simulink model "Marine_LocoMotive_UAV_est_git"  (R2018a)
settings: Solver=ode4  StartTime=0.0  StopTime=40  FixedStep=T  MaxStep=2*T  MinStep=T  RelTol=1e-4
values from neighbouring files (symbols this model uses):
  a_11 = 0.05*m_b    (= 0.625)    [Marine_LocoMotive_UAV_est_git_parameters.m]    (also in Marine_LocoMotive_UAV_medium_est_git_parameters.m = 1.6875; heave_dynamics_chart.m)
  a_33 = m_b    (= 12.5)    [Marine_LocoMotive_UAV_est_git_parameters.m]    (also in Marine_LocoMotive_UAV_medium_est_git_parameters.m = 33.75; heave_dynamics_chart.m)
  A_w = 1*3.3/2    (= 1.65)    [Marine_LocoMotive_UAV_est_git_parameters.m]    (also in Marine_LocoMotive_UAV_medium_est_git_parameters.m = 0.6)
  A_w2 = 1*1.2/2    (= 0.6)    [Marine_LocoMotive_UAV_est_git_parameters.m]    (also in Marine_LocoMotive_UAV_medium_est_git_parameters.m = 0.305)
  Ac = 0.0331    [Marine_LocoMotive_UAV_est_git_parameters.m]    (also in Marine_LocoMotive_UAV_medium_est_git_parameters.m = 0.422)
  alpha_bar = pi/4    (= 0.785398163397)    [Marine_LocoMotive_UAV_est_git_parameters.m]    (also in Marine_LocoMotive_UAV_medium_est_git_parameters.m; heave_dynamics_chart.m = pi/4*sign(V_bar(j)))
  Am = sysd.denominator{1}    [Marine_LocoMotive_UAV_est_git_parameters.m]    (also in Marine_LocoMotive_UAV_medium_est_git_parameters.m)
  Am1_LPF = sysd.denominator{1}    [Marine_LocoMotive_UAV_est_git_parameters.m]    (also in Marine_LocoMotive_UAV_medium_est_git_parameters.m)
  Am2_LPF = sysd.denominator{1}    [Marine_LocoMotive_UAV_est_git_parameters.m]    (also in Marine_LocoMotive_UAV_medium_est_git_parameters.m)
  Am_asw_LPF = sysd.denominator{1}    [Marine_LocoMotive_UAV_est_git_parameters.m]    (also in Marine_LocoMotive_UAV_medium_est_git_parameters.m)
  Am_coup_LPF = sysd.denominator{1}    [Marine_LocoMotive_UAV_est_git_parameters.m]    (also in Marine_LocoMotive_UAV_medium_est_git_parameters.m)
  Am_fast_coup_LPF = sysd.denominator{1}    [Marine_LocoMotive_UAV_est_git_parameters.m]    (also in Marine_LocoMotive_UAV_medium_est_git_parameters.m)
  Am_rdeL_LPF = sysd.denominator{1}    [Marine_LocoMotive_UAV_est_git_parameters.m]    (also in Marine_LocoMotive_UAV_medium_est_git_parameters.m)
  Am_reL_LPF = sysd.denominator{1}    [Marine_LocoMotive_UAV_est_git_parameters.m]    (also in Marine_LocoMotive_UAV_medium_est_git_parameters.m)
  Am_rref20_LPF = sysd.denominator{1}    [Marine_LocoMotive_UAV_est_git_parameters.m]    (also in Marine_LocoMotive_UAV_medium_est_git_parameters.m)
  Am_rref_LPF = sysd.denominator{1}    [Marine_LocoMotive_UAV_est_git_parameters.m]    (also in Marine_LocoMotive_UAV_medium_est_git_parameters.m)
  AmAlpha_LPF = sysd.denominator{1}    [Marine_LocoMotive_UAV_est_git_parameters.m]    (also in Marine_LocoMotive_UAV_medium_est_git_parameters.m)
  Amp_sf = 3    [Marine_LocoMotive_UAV_est_git_parameters.m]    (also in Marine_LocoMotive_UAV_medium_est_git_parameters.m)
  Amp_sf_rp = 0.05*m_u*g    (= 0.8829)    [Marine_LocoMotive_UAV_est_git_parameters.m]    (also in Marine_LocoMotive_UAV_medium_est_git_parameters.m = 9.56475)
  AmV_LPF = sysd.denominator{1}    [Marine_LocoMotive_UAV_est_git_parameters.m]    (also in Marine_LocoMotive_UAV_medium_est_git_parameters.m)
  AmZ_LPF = sysd.denominator{1}    [Marine_LocoMotive_UAV_est_git_parameters.m]    (also in Marine_LocoMotive_UAV_medium_est_git_parameters.m)
  b_11 = 0    [Marine_LocoMotive_UAV_est_git_parameters.m]    (also in Marine_LocoMotive_UAV_medium_est_git_parameters.m; heave_dynamics_chart.m)
  b_33 = 2*m_b*omega_h    (= 19.6349540849)    [Marine_LocoMotive_UAV_est_git_parameters.m]    (also in Marine_LocoMotive_UAV_medium_est_git_parameters.m = 84.8230016469; buoyancy_calc.m = 4.18879020479; heave_dynamics_chart.m = 2*m_b*omega_h)
  Bm = sysd.numerator{1}    [Marine_LocoMotive_UAV_est_git_parameters.m]    (also in Marine_LocoMotive_UAV_medium_est_git_parameters.m)
  Bm1_LPF = sysd.numerator{1}    [Marine_LocoMotive_UAV_est_git_parameters.m]    (also in Marine_LocoMotive_UAV_medium_est_git_parameters.m)
  Bm2_LPF = sysd.numerator{1}    [Marine_LocoMotive_UAV_est_git_parameters.m]    (also in Marine_LocoMotive_UAV_medium_est_git_parameters.m)
  Bm_asw_LPF = sysd.numerator{1}    [Marine_LocoMotive_UAV_est_git_parameters.m]    (also in Marine_LocoMotive_UAV_medium_est_git_parameters.m)
  Bm_coup_LPF = sysd.numerator{1}    [Marine_LocoMotive_UAV_est_git_parameters.m]    (also in Marine_LocoMotive_UAV_medium_est_git_parameters.m)
  Bm_fast_coup_LPF = sysd.numerator{1}    [Marine_LocoMotive_UAV_est_git_parameters.m]    (also in Marine_LocoMotive_UAV_medium_est_git_parameters.m)
  Bm_rdeL_LPF = sysd.numerator{1}    [Marine_LocoMotive_UAV_est_git_parameters.m]    (also in Marine_LocoMotive_UAV_medium_est_git_parameters.m)
  Bm_reL_LPF = sysd.numerator{1}    [Marine_LocoMotive_UAV_est_git_parameters.m]    (also in Marine_LocoMotive_UAV_medium_est_git_parameters.m)
  Bm_rref20_LPF = sysd.numerator{1}    [Marine_LocoMotive_UAV_est_git_parameters.m]    (also in Marine_LocoMotive_UAV_medium_est_git_parameters.m)
  Bm_rref_LPF = sysd.numerator{1}    [Marine_LocoMotive_UAV_est_git_parameters.m]    (also in Marine_LocoMotive_UAV_medium_est_git_parameters.m)
  BmAlpha_LPF = sysd.numerator{1}    [Marine_LocoMotive_UAV_est_git_parameters.m]    (also in Marine_LocoMotive_UAV_medium_est_git_parameters.m)
  BmV_LPF = sysd.numerator{1}    [Marine_LocoMotive_UAV_est_git_parameters.m]    (also in Marine_LocoMotive_UAV_medium_est_git_parameters.m)
  BmZ_LPF = sysd.numerator{1}    [Marine_LocoMotive_UAV_est_git_parameters.m]    (also in Marine_LocoMotive_UAV_medium_est_git_parameters.m)
  C_S = [5;9]*10^-3    [Marine_LocoMotive_UAV_est_git_parameters.m]    (also in Marine_LocoMotive_UAV_medium_est_git_parameters.m; heave_dynamics_chart.m = 0.075/(log10(Re)-2)^2)
  Cd_u = 0.2    [Marine_LocoMotive_UAV_est_git_parameters.m]    (also in Marine_LocoMotive_UAV_medium_est_git_parameters.m)
  D_x = b_11 + D_s(1)    [Marine_LocoMotive_UAV_est_git_parameters.m]    (also in Marine_LocoMotive_UAV_medium_est_git_parameters.m; heave_dynamics_chart.m = b_11 + D_s(i,j))
  D_z = b_33 + D_s(2)    [Marine_LocoMotive_UAV_est_git_parameters.m]    (also in Marine_LocoMotive_UAV_medium_est_git_parameters.m; heave_dynamics_chart.m)
  dc_M_p = 6.7    [Marine_LocoMotive_UAV_est_git_parameters.m]    (also in Marine_LocoMotive_UAV_medium_est_git_parameters.m)
  Delta_h = (A_im/A_b-0.5)*h_b    (= -0.0625)    [Marine_LocoMotive_UAV_est_git_parameters.m]    (also in Marine_LocoMotive_UAV_medium_est_git_parameters.m = -0.075; heave_dynamics_chart.m)
  eps_V = 0.1    [Marine_LocoMotive_UAV_est_git_parameters.m]    (also in Marine_LocoMotive_UAV_medium_est_git_parameters.m)
  epsilon_1 = 5    [Marine_LocoMotive_UAV_est_git_parameters.m]    (also in Marine_LocoMotive_UAV_medium_est_git_parameters.m)
  epsilon_e_u1 = 0.05    [Marine_LocoMotive_UAV_est_git_parameters.m]    (also in Marine_LocoMotive_UAV_medium_est_git_parameters.m)
  epsilon_w = 0    [Marine_LocoMotive_UAV_est_git_parameters.m]    (also in Marine_LocoMotive_UAV_medium_est_git_parameters.m)
  epsilon_w2 = pi    (= 3.14159265359)    [Marine_LocoMotive_UAV_est_git_parameters.m]    (also in Marine_LocoMotive_UAV_medium_est_git_parameters.m)
  g = 9.81    [Marine_LocoMotive_UAV_est_git_parameters.m]    (also in Marine_LocoMotive_UAV_medium_est_git_parameters.m; heave_dynamics_chart.m)
  gamma_d_p = (2*0.3/0.03*2*0.2*12/4)/10    (= 2.4)    [Marine_LocoMotive_UAV_est_git_parameters.m]    (also in Marine_LocoMotive_UAV_medium_est_git_parameters.m)
  H = 10    [Marine_LocoMotive_UAV_est_git_parameters.m]    (also in Marine_LocoMotive_UAV_medium_est_git_parameters.m)
  h_b = 0.25    [Marine_LocoMotive_UAV_est_git_parameters.m]    (also in Marine_LocoMotive_UAV_medium_est_git_parameters.m = 0.3; buoyancy_calc.m = 0.15; heave_dynamics_chart.m)
  J_b = m_b*h_b*l_b/12    (= 0.208333333333)    [Marine_LocoMotive_UAV_est_git_parameters.m]    (also in Marine_LocoMotive_UAV_medium_est_git_parameters.m = 1.265625; heave_dynamics_chart.m)
  J_u = 0.03    [Marine_LocoMotive_UAV_est_git_parameters.m]    (also in Marine_LocoMotive_UAV_medium_est_git_parameters.m = 1.51708333333)
  K = 40    [Marine_LocoMotive_UAV_est_git_parameters.m]    (also in Marine_LocoMotive_UAV_medium_est_git_parameters.m = 83.3333333333)
  k3 = 24    [Marine_LocoMotive_UAV_est_git_parameters.m]    (also in Marine_LocoMotive_UAV_medium_est_git_parameters.m)
  k4 = 0.8    [Marine_LocoMotive_UAV_est_git_parameters.m]    (also in Marine_LocoMotive_UAV_medium_est_git_parameters.m)
  k_w = omega_w^2/g    (= 0.0628797426165)    [Marine_LocoMotive_UAV_est_git_parameters.m]    (also in Marine_LocoMotive_UAV_medium_est_git_parameters.m = 0.160972141098; heave_dynamics_chart.m = omega_w^2/g)
  k_w2 = omega_w2^2/g    (= 0.160972141098)    [Marine_LocoMotive_UAV_est_git_parameters.m]    (also in Marine_LocoMotive_UAV_medium_est_git_parameters.m = 0.251518970466)
  kd_a = 5.6    [Marine_LocoMotive_UAV_est_git_parameters.m]    (also in Marine_LocoMotive_UAV_medium_est_git_parameters.m)
  kd_r = 19.5    [Marine_LocoMotive_UAV_est_git_parameters.m]    (also in Marine_LocoMotive_UAV_medium_est_git_parameters.m)
  kd_t = 10    [Marine_LocoMotive_UAV_est_git_parameters.m]    (also in Marine_LocoMotive_UAV_medium_est_git_parameters.m = 25)
  kd_x = 5    [Marine_LocoMotive_UAV_est_git_parameters.m]    (also in Marine_LocoMotive_UAV_medium_est_git_parameters.m)
  kd_z = 2    [Marine_LocoMotive_UAV_est_git_parameters.m]    (also in Marine_LocoMotive_UAV_medium_est_git_parameters.m)
  ki_a = 1.6    [Marine_LocoMotive_UAV_est_git_parameters.m]    (also in Marine_LocoMotive_UAV_medium_est_git_parameters.m)
  ki_r = 9    [Marine_LocoMotive_UAV_est_git_parameters.m]    (also in Marine_LocoMotive_UAV_medium_est_git_parameters.m)
  ki_T = 12    [Marine_LocoMotive_UAV_est_git_parameters.m]    (also in Marine_LocoMotive_UAV_medium_est_git_parameters.m)
  ki_x = 1.2    [Marine_LocoMotive_UAV_est_git_parameters.m]    (also in Marine_LocoMotive_UAV_medium_est_git_parameters.m)
  ki_z = 1    [Marine_LocoMotive_UAV_est_git_parameters.m]    (also in Marine_LocoMotive_UAV_medium_est_git_parameters.m)
  kp_a = 9.6    [Marine_LocoMotive_UAV_est_git_parameters.m]    (also in Marine_LocoMotive_UAV_medium_est_git_parameters.m)
  kp_r = 45    [Marine_LocoMotive_UAV_est_git_parameters.m]    (also in Marine_LocoMotive_UAV_medium_est_git_parameters.m)
  kp_t = 20    [Marine_LocoMotive_UAV_est_git_parameters.m]    (also in Marine_LocoMotive_UAV_medium_est_git_parameters.m = 50)
  kp_T = 25    [Marine_LocoMotive_UAV_est_git_parameters.m]    (also in Marine_LocoMotive_UAV_medium_est_git_parameters.m)
  kp_x = 7    [Marine_LocoMotive_UAV_est_git_parameters.m]    (also in Marine_LocoMotive_UAV_medium_est_git_parameters.m)
  kp_z = 3    [Marine_LocoMotive_UAV_est_git_parameters.m]    (also in Marine_LocoMotive_UAV_medium_est_git_parameters.m)
  L = 0.2    [Marine_LocoMotive_UAV_est_git_parameters.m]    (also in Marine_LocoMotive_UAV_medium_est_git_parameters.m = 0.8)
  l_b = 0.8    [Marine_LocoMotive_UAV_est_git_parameters.m]    (also in Marine_LocoMotive_UAV_medium_est_git_parameters.m = 1.5; buoyancy_calc.m = 0.5; heave_dynamics_chart.m)
  Lc_0 = 7    [Marine_LocoMotive_UAV_est_git_parameters.m]    (also in Marine_LocoMotive_UAV_medium_est_git_parameters.m = 20)
  LIMIT_CMD_PITCH = 45*pi/180    (= 0.785398163397)    [Marine_LocoMotive_UAV_est_git_parameters.m]    (also in Marine_LocoMotive_UAV_medium_est_git_parameters.m)
  LIMIT_uCMD_HEIGHT = 0.9*n_motors*K    (= 144)    [Marine_LocoMotive_UAV_est_git_parameters.m]    (also in Marine_LocoMotive_UAV_medium_est_git_parameters.m = 450)
  m_b = rho_w*Vol_b/4    (= 12.5)    [Marine_LocoMotive_UAV_est_git_parameters.m]    (also in Marine_LocoMotive_UAV_medium_est_git_parameters.m = 33.75; buoyancy_calc.m = 5; heave_dynamics_chart.m)
  m_u = 1.8    [Marine_LocoMotive_UAV_est_git_parameters.m]    (also in Marine_LocoMotive_UAV_medium_est_git_parameters.m = 19.5)
  min_sf = 5    [Marine_LocoMotive_UAV_est_git_parameters.m]    (also in Marine_LocoMotive_UAV_medium_est_git_parameters.m)
  min_sf_rp = 0.35*m_u*g    (= 6.1803)    [Marine_LocoMotive_UAV_est_git_parameters.m]    (also in Marine_LocoMotive_UAV_medium_est_git_parameters.m = 66.95325)
  n_motors = 4    [Marine_LocoMotive_UAV_est_git_parameters.m]    (also in Marine_LocoMotive_UAV_medium_est_git_parameters.m = 6)
  nu_w = 1.787*10^-6    (= 1.787e-06)    [Marine_LocoMotive_UAV_est_git_parameters.m]    (also in Marine_LocoMotive_UAV_medium_est_git_parameters.m; buoyancy_calc.m; heave_dynamics_chart.m)
  omega_w = 2*pi/T_w    (= 0.785398163397)    [Marine_LocoMotive_UAV_est_git_parameters.m]    (also in Marine_LocoMotive_UAV_medium_est_git_parameters.m = 1.25663706144; heave_dynamics_chart.m = 2*pi/T_i)
  omega_w2 = 2*pi/T_w2    (= 1.25663706144)    [Marine_LocoMotive_UAV_est_git_parameters.m]    (also in Marine_LocoMotive_UAV_medium_est_git_parameters.m = 1.57079632679)
  r_0 = sqrt( (X0_b(1) - X0_u(1))^2 +(X0_b(2) - X0_u(2))^2 )    [Marine_LocoMotive_UAV_est_git_parameters.m]    (also in Marine_LocoMotive_UAV_medium_est_git_parameters.m)
  R_b = 0.1    [buoyancy_calc.m]
  r_bar = Lc_0-0.3    (= 6.7)    [Marine_LocoMotive_UAV_est_git_parameters.m]    (also in Marine_LocoMotive_UAV_medium_est_git_parameters.m = 19.7)
  r_min = (zu_bar-H)-0.2    [Marine_LocoMotive_UAV_est_git_parameters.m]    (also in Marine_LocoMotive_UAV_medium_est_git_parameters.m)
  rho_a = 1.225    [Marine_LocoMotive_UAV_est_git_parameters.m]    (also in Marine_LocoMotive_UAV_medium_est_git_parameters.m)
  rho_w = 1000    [Marine_LocoMotive_UAV_est_git_parameters.m]    (also in Marine_LocoMotive_UAV_medium_est_git_parameters.m; buoyancy_calc.m; heave_dynamics_chart.m)
  T = 1/500    (= 0.002)    [Marine_LocoMotive_UAV_est_git_parameters.m]    (also in Marine_LocoMotive_UAV_medium_est_git_parameters.m)
  T_init = 10    [Marine_LocoMotive_UAV_est_git_parameters.m]    (also in Marine_LocoMotive_UAV_medium_est_git_parameters.m)
  Theta0 = 0    [Marine_LocoMotive_UAV_est_git_parameters.m]    (also in Marine_LocoMotive_UAV_medium_est_git_parameters.m)
  torque_corr = 2*cosd(60)+1    [Marine_LocoMotive_UAV_est_git_parameters.m]    (also in Marine_LocoMotive_UAV_medium_est_git_parameters.m)
  u_s = w_dir*A_w^2*omega_w*k_w*exp(2*k_w*(-Delta_h/2))    [Marine_LocoMotive_UAV_est_git_parameters.m]    (also in Marine_LocoMotive_UAV_medium_est_git_parameters.m)
  u_s2 = w_dir2*A_w2^2*omega_w2*k_w2*exp(2*k_w2*(-Delta_h/2))    [Marine_LocoMotive_UAV_est_git_parameters.m]    (also in Marine_LocoMotive_UAV_medium_est_git_parameters.m)
  u_t = -1*0.5*1    (= -0.5)    [Marine_LocoMotive_UAV_est_git_parameters.m]    (also in Marine_LocoMotive_UAV_medium_est_git_parameters.m)
  u_w = 0*0.2    (= 0)    [Marine_LocoMotive_UAV_est_git_parameters.m]    (also in Marine_LocoMotive_UAV_medium_est_git_parameters.m)
  V0_b = [u_t+u_w+u_s+v_x_w, v_z_w].*[1 1]    [Marine_LocoMotive_UAV_est_git_parameters.m]    (also in Marine_LocoMotive_UAV_medium_est_git_parameters.m = [u_t+u_w+u_s+v_x_w, v_z_w])
  V0_u = V0_b    [Marine_LocoMotive_UAV_est_git_parameters.m]    (also in Marine_LocoMotive_UAV_medium_est_git_parameters.m = [0 0])
  V_bar = 4    [Marine_LocoMotive_UAV_est_git_parameters.m]    (also in Marine_LocoMotive_UAV_medium_est_git_parameters.m; heave_dynamics_chart.m = [-20:0.1:20]')
  Vol_b = A_b*l_b    (= 0.05)    [Marine_LocoMotive_UAV_est_git_parameters.m]    (also in Marine_LocoMotive_UAV_medium_est_git_parameters.m = 0.135; heave_dynamics_chart.m)
  w_dir = 1    [Marine_LocoMotive_UAV_est_git_parameters.m]    (also in Marine_LocoMotive_UAV_medium_est_git_parameters.m; heave_dynamics_chart.m)
  w_dir2 = 1    [Marine_LocoMotive_UAV_est_git_parameters.m]    (also in Marine_LocoMotive_UAV_medium_est_git_parameters.m)
  X0_b = [0,H-Delta_h]    [Marine_LocoMotive_UAV_est_git_parameters.m]    (also in Marine_LocoMotive_UAV_medium_est_git_parameters.m)
  X0_u = X0_b + [3/7 3/7]*Lc_0    [Marine_LocoMotive_UAV_est_git_parameters.m]    (also in Marine_LocoMotive_UAV_medium_est_git_parameters.m)
  zu_bar = X0_b(2) + Lc_0*sin(alpha_bar_0)    [Marine_LocoMotive_UAV_est_git_parameters.m]    (also in Marine_LocoMotive_UAV_medium_est_git_parameters.m)
undefined symbols (not defined in the file or in its folder): Am_HPF, Am_LPF, Am_LPF2, an1, an1_v, an2, an3, Bm_HPF, Bm_LPF, Bm_LPF2, bn1, bn1_v, bn2, bn3, DiscIntNeverNeededParam, F, Light, magnitude, MIL, OMEGA_FILTER_OUTER, Tc, Tg, Tn, Ts, Tsc, Tz, X_GPS_offset
libraries: simulink x55, simulink_extras x9, aerolibwind2 x2
(part 3 of 9)

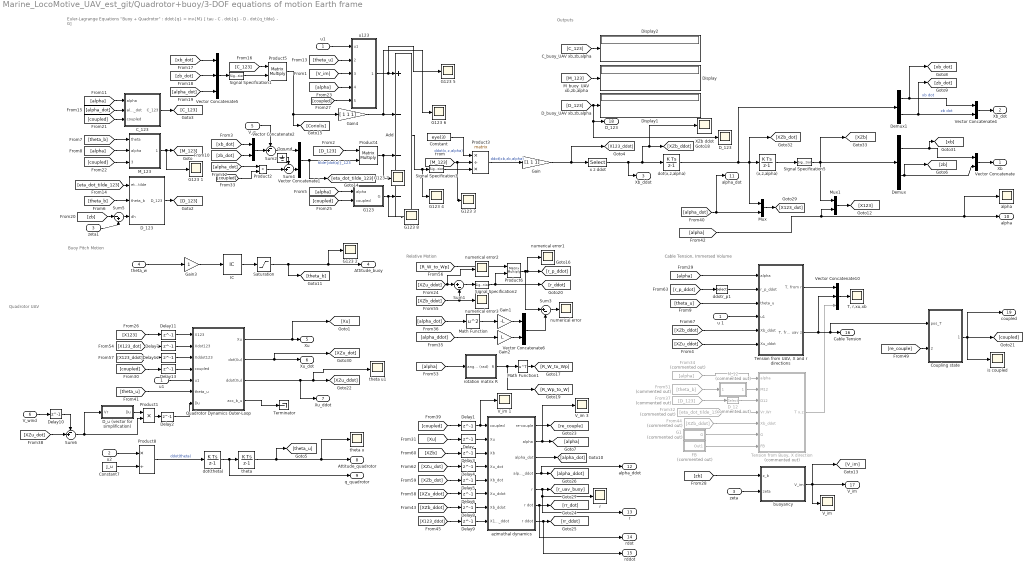
== system Marine_LocoMotive_UAV_est_git/Quadrotor+buoy/3-DOF equations of motion Earth frame ==
  note: Relative Motion
  note: Outputs
  note: Buoy Pitch Motion
  note: Cable Tension, Immersed Volume
  note: Quadrotor UAV
  note: Euler-Lagrange Equations "Buoy + Quadrotor" : ddot{q} = inv{M} [ tau - C . dot{q} - D . dot{q_tilde} - G]
  u1 : Inport
  u2 : Inport  Port=2
  zeta : Inport  Port=3
  theta_w : Inport  Port=4
  V_w : Inport  Port=5
  V_wind : Inport  Port=6
  "  r   " : Scope
  (x,z,alpha) : DiscreteIntegrator  InitialCondition=[pos_b_ini]  SampleTime=-1  ICPrevOutput=DiscIntNeverNeededParam  ICPrevScaledInput=DiscIntNeverNeededParam
  Add : Sum  Inputs=+---
  C_123 : Subsystem
  Constant : Constant  Value=eye(3)
  Constant7 : Constant  Value=J_u
  Coupling state : Subsystem
  D_12 : Selector  Commented=on  NumberOfDimensions=2  InputPortWidth=3  IndexOptions=Starting index (dialog),Starting index (dialog)  Indices=1,1  OutputSizes=2,2
  D_123 : Subsystem
  "D_123   " : Scope
  D_u (vector for simplification) : Subsystem
  Delay{,1,3..9,11..13} (12 alike) : Delay  DelayLength=1
  Delay10 : Delay  DelayLength=1  InitialCondition=[0 0]
  Delay2 : Delay  DelayLength=1  InitialCondition=[0 0]
  Demux : Demux  Outputs=2
  Demux1 : Demux  Outputs=2
  Display : Display
  Display1 : Display
  Display2 : Display
  FB : Subsystem  Commented=on
  From32 : From  Commented=on  GotoTag=eta_dot_tilde_12
  From34 : From  Commented=on  GotoTag=alpha
  From37 : From  Commented=on  GotoTag=D_123
  From44 : From  Commented=on  GotoTag=XZb_ddot
  From51 : From  Commented=on  GotoTag=theta_b
  G1 : Subsystem  Commented=on
  G123 : Subsystem
  G123 {1..8} (8 alike) : Scope
  Gain : Gain  Gain=[1 1 1]
  Gain1 : Gain  Gain=-L
  Gain2 : Gain  Gain=L
  Gain3 : Gain
  Gain4 : Gain  Gain=[ 1 1 1]
  Ground : Ground
  IC : InitialCondition  Value=0
  M_12 : Subsystem  Commented=on
  M_123 : Subsystem
  Math Function : Math  Operator=square  SaturateOnIntegerOverflow=on
  Math Function1 : Math  Operator=transpose  SaturateOnIntegerOverflow=on
  Mux : Mux  Inputs=2
  Mux1 : Mux  Inputs=2
  Product1 : Product  Inputs=**  SaturateOnIntegerOverflow=on  InputSameDT=on  OutDataTypeStr=Inherit: Same as first input
  Product2 : Product  Inputs=**  SaturateOnIntegerOverflow=on  InputSameDT=on  OutDataTypeStr=Inherit: Same as first input
  Product3 : Product  Inputs=*/*  Multiplication=Matrix(*)  SaturateOnIntegerOverflow=on  InputSameDT=on  OutDataTypeStr=Inherit: Same as first input
  Product4 : Product  Inputs=**  Multiplication=Matrix(*)  SaturateOnIntegerOverflow=on  InputSameDT=on  OutDataTypeStr=Inherit: Same as first input
  Product5 : Product  Inputs=**  Multiplication=Matrix(*)  SaturateOnIntegerOverflow=on  InputSameDT=on  OutDataTypeStr=Inherit: Same as first input
  Product6 : Product  Multiplication=Matrix(*)
  Product8 : Product  Inputs=*/  SaturateOnIntegerOverflow=on  InputSameDT=on  OutDataTypeStr=Inherit: Same as first input
  Quadrotor Dynamics Outer-Loop : Subsystem
  Saturation : Saturate  UpperLimit=0.15  LowerLimit=-0.15
  Signal Specification1 : SignalSpecification  Dimensions=3
  Signal Specification2 : SignalSpecification  Dimensions=2
  Signal Specification3 : SignalSpecification  Dimensions=3
  Signal Specification5 : SignalSpecification  Dimensions=2
  Sum1 : Sum  Inputs=|+-
  Sum2 : Sum  Inputs=-+|  SaturateOnIntegerOverflow=on
  Sum3 : Sum  Inputs=|+-
  Sum4 : Sum  Inputs=-+|  SaturateOnIntegerOverflow=on
  Sum5 : Sum  Inputs=|-+  SaturateOnIntegerOverflow=on
  Sum6 : Sum  Inputs=-+|  SaturateOnIntegerOverflow=on
  "T, r,xu,xb" : Scope
  "Tension from Buoy, X direction" : Subsystem  Commented=on
  "Tension from UAV, X and r directions" : Subsystem
  Terminator : Terminator
  "V_im " : Scope
  V_im 1 : Scope
  V_im 3 : Scope
  Vector Concatenate{,1..2,4,6} (5 alike) : Concatenate
  Vector Concatenate10 : Concatenate  NumInputs=3
  Vector Concatenate5 : Concatenate  NumInputs=3
  "XZb ddot " : Scope
  "alpha  " : Scope
  azimuthal dynamics : Subsystem
  buoyancy : Subsystem
  ddotr_p1 : Selector  InputPortWidth=2  IndexOptions=Index vector (dialog)  Indices=1  OutputSizes=2
  dot(theta) : DiscreteIntegrator  gainval=1  InitialCondition=q_b_ini  SampleTime=-1  ICPrevOutput=DiscIntNeverNeededParam  ICPrevScaledInput=DiscIntNeverNeededParam
  dot(x,z,alpha) : DiscreteIntegrator  InitialCondition=[v_b_ini]  SampleTime=-1  ICPrevOutput=DiscIntNeverNeededParam  ICPrevScaledInput=DiscIntNeverNeededParam
  "is coupled " : Scope
  numerical error{,1..3} (4 alike) : Scope
  "rotation matrix R " : Subsystem
  theta : DiscreteIntegrator  InitialCondition=theta_q_ini  SampleTime=-1  StateName=theta  ICPrevOutput=DiscIntNeverNeededParam  ICPrevScaledInput=DiscIntNeverNeededParam
  theta u : Scope
  theta u1 : Scope
  u 1 : InportShadow
  "u1  " : InportShadow
  u123 : Subsystem
  x z ddot : Selector  InputPortWidth=3  IndexOptions=Index vector (dialog)  Indices=[1 2]  OutputSizes=1
  zeta1 : InportShadow  Port=3
  Xb : Outport  Unit=m  InitialOutput=0
  Xb_dot : Outport  Port=2  Unit=m  InitialOutput=0
  Xb_ddot : Outport  Port=3  Unit=m  InitialOutput=0
  Attitude_buoy : Outport  Port=4  Unit=rad/s^2  InitialOutput=0
  Xu : Outport  Port=5  Unit=m  InitialOutput=0
  Xu_dot : Outport  Port=6  Unit=m/s  InitialOutput=0
  Xu_ddot : Outport  Port=7  Unit=m/s  InitialOutput=0
  Attitude_quadrotor : Outport  Port=8  Unit=rad  InitialOutput=0
  q_quadrotor : Outport  Port=9  Unit=rad/s  InitialOutput=0
  alpha : Outport  Port=10  Unit=m  InitialOutput=0
  alpha_dot : Outport  Port=11  Unit=m  InitialOutput=0
  alpha_ddot : Outport  Port=12  Unit=m  InitialOutput=0
  "  r" : Outport  Port=13  Unit=m  InitialOutput=0
  "  rdot" : Outport  Port=14  Unit=m  InitialOutput=0
  "  rddot" : Outport  Port=15  Unit=m  InitialOutput=0
  Cable Tension : Outport  Port=16  Unit=rad/s^2  InitialOutput=0
  V_im : Outport  Port=17  Unit=m  InitialOutput=0
  "D_123 " : Outport  Port=18  Unit=m  InitialOutput=0
  coupled : Outport  Port=19  Unit=m  InitialOutput=0
  wires:
  u123/1(u123) -> G123 5/1, Add/1
  Product4/1 -> G123 7/1, Add/3
  [D_123] -> Product4/1
  Vector Concatenate1/1 -> [eta_dot_tilde_123], Product4/2  "tilde{dot(q)}_123"
  G123/1(G) -> G123 8/1, Add/4
  [alpha] -> Mux1/2, "alpha  "/1, alpha/1
  [theta_b] -> D_123/2(theta_b)
  D_123/1(D_123) -> [D_123]
  [theta_b] -> M_123/1(theta)
  [alpha] -> M_123/2(alpha)
  Demux1/2 -> [zb_dot], Vector Concatenate4/2  "zb dot"
  Demux1/1 -> [xb_dot], Vector Concatenate4/1  "xb dot"
  [xb_dot] -> Vector Concatenate2/1
  [zb_dot] -> Vector Concatenate2/2
  Vector Concatenate2/1 -> Sum2/2
  V_w/1 -> Sum2/1
  Sum2/1 -> Vector Concatenate1/1
  Sum4/1 -> Vector Concatenate1/2
  theta_w/1 -> Gain3/1
  dot(theta)/1 -> q_quadrotor/1, theta/1
  theta/1 -> [theta_u], theta u/1, Attitude_quadrotor/1
  Constant7/1 -> Product8/2
  u2/1 -> Product8/1
  [theta_u] -> u123/2(theta)
  [V_im] -> u123/3(V_im)
  [alpha] -> G123/1(alpha)
  Demux/1 -> [xb], Vector Concatenate/1
  Demux/2 -> [zb], Vector Concatenate/2
  M_123/1(M_123) -> G123 1/1, [M_123]
  Product8/1 -> dot(theta)/1  "ddot(theta)"
  [M_123] -> G123 3/1, Product3/2
  Constant/1 -> Product3/1  "ddot(x,z,alpha)"
  Product3/1 -> Gain/1  "ddot(xb,zb,alpha)"
  IC/1 -> Saturation/1
  [alpha] -> C_123/1("alpha ")
  [alpha_dot] -> C_123/2(alpha_dot)
  C_123/1(C_123) -> [C_123]
  Vector Concatenate5/1 -> Signal Specification1/1
  [xb_dot] -> Vector Concatenate5/1
  [zb_dot] -> Vector Concatenate5/2
  [alpha_dot] -> Vector Concatenate5/3
  [C_123] -> Product5/1
  Product5/1 -> [Coriolis], Gain4/1
  Gain/1 -> [X123_ddot], x z ddot/1
  [alpha] -> u123/4(alpha)
  [r_p_ddot] -> ddotr_p1/1
  [theta_u] -> "Tension from UAV, X and r directions"/3(theta_u)
  u 1/1 -> "Tension from UAV, X and r directions"/4(u1)
  [D_123] -> "D_123 "/1, "D_123   "/1, Display1/1
  [M_123] -> Display/1
  [C_123] -> Display2/1
  (x,z,alpha)/1 -> Signal Specification5/1
  [zb] -> buoyancy/1(z_b)
  zeta/1 -> buoyancy/2(zeta)
  From34/1 -> "Tension from Buoy, X direction"/1(alpha)
  D_12/1 -> "Tension from Buoy, X direction"/3(D12)
  buoyancy/1(V_im) -> "V_im "/1, V_im/1, [V_im]
  M_12/1(M_12) -> "Tension from Buoy, X direction"/2(M12)
  From37/1 -> D_12/1
  From44/1 -> "Tension from Buoy, X direction"/5(Xb_ddot)
  From32/1 -> "Tension from Buoy, X direction"/4(Vr,Wr)
  [XZb_ddot] -> "Tension from UAV, X and r directions"/5(Xb_ddot)
  G1/1(G) -> "Tension from Buoy, X direction"/6(G)
  From51/1 -> M_12/1(theta)
  x z ddot/1 -> Xb_ddot/1, "XZb ddot "/1, [XZb_ddot], dot(x,z,alpha)/1
  ddotr_p1/1 -> "Tension from UAV, X and r directions"/2(r_p_ddot)
  [XZu_ddot] -> "Tension from UAV, X and r directions"/6(Xu_ddot)
  FB/1(Out1) -> "Tension from Buoy, X direction"/7(FB)
  Vector Concatenate10/1 -> "T, r,xu,xb"/1
  "Tension from Buoy, X direction"/1(T x,z) -> Vector Concatenate10/3
  Gain2/1 -> Vector Concatenate6/2
  [R_W_to_Wp] -> Product6/1
  Vector Concatenate6/1 -> Sum3/2
  "rotation matrix R "/1(R) -> [R_Wp_to_W], Math Function1/1
  Product6/1 -> Sum3/1, numerical error1/1, [r_p_ddot]
  Gain1/1 -> Vector Concatenate6/1
  Math Function/1 -> Gain1/1
  Sum1/1 -> Signal Specification2/1
  [XZu_ddot] -> numerical error2/1, Sum1/1
  Math Function1/1 -> [R_W_to_Wp]
  Sum3/1 -> numerical error/1
  [XZb_ddot] -> numerical error3/1, Sum1/2
  [alpha] -> "rotation matrix R "/1(angle (rad))
  [alpha_dot] -> Math Function/1
  Saturation/1 -> G123 2/1, Attitude_buoy/1, [theta_b]
  Add/1 -> G123 4/1, Signal Specification3/1
  Gain3/1 -> IC/1
  Gain4/1 -> G123 6/1, Add/2
  Product2/1 -> Sum4/2
  Ground/1 -> Sum4/1
  [eta_dot_tilde_123] -> D_123/1(eta_dot_tilde)
  Sum5/1 -> D_123/3(dh)
  [zb] -> Sum5/1
  zeta1/1 -> Sum5/2
  [coupled] -> C_123/3(coupled)
  [coupled] -> M_123/3(coupled)
  [coupled] -> G123/2(coupled)
  u1/1 -> u123/1(u1)
  Signal Specification1/1 -> Product5/2
  Signal Specification2/1 -> Product6/2, [r_ddot]
  Signal Specification3/1 -> Product3/3
  Signal Specification5/1 -> [XZb], Mux1/1, Demux/1
  Quadrotor Dynamics Outer-Loop/1(Xu) -> Xu/1, [Xu]
  [coupled] -> Delay13/1
  "u1  "/1 -> Quadrotor Dynamics Outer-Loop/5(u1)
  [theta_u] -> Quadrotor Dynamics Outer-Loop/6(theta_u)
  Quadrotor Dynamics Outer-Loop/2(dot(Xu)) -> [XZu_dot], Xu_dot/1
  Product1/1 -> Delay2/1
  [coupled] -> u123/5(coupled)
  [alpha_dot] -> Product2/1
  [coupled] -> Product2/2
  [Xu] -> Delay/1
  azimuthal dynamics/1(re-couple) -> [re_couple]
  azimuthal dynamics/2(alpha) -> V_im 3/1, [alpha]
  azimuthal dynamics/3("alpha_dot ") -> [alpha_dot]
  azimuthal dynamics/4(alpha_ddot) -> alpha_ddot/1, [alpha_ddot]
  Delay/1 -> azimuthal dynamics/2(Xu)
  azimuthal dynamics/5("r ") -> "  r"/1, "  r   "/1, [r_uav_buoy]
  [X123] -> Delay11/1
  Delay3/1 -> azimuthal dynamics/3(Xb)
  [X123_ddot] -> Delay12/1
  [X123_dot] -> Delay7/1
  dot(x,z,alpha)/1 -> Mux/1, (x,z,alpha)/1, [XZb_dot], Demux1/1
  [alpha_dot] -> alpha_dot/1, Mux/2
  Mux/1 -> [X123_dot]
  Mux1/1 -> [X123]
  Vector Concatenate4/1 -> Xb_dot/1
  Vector Concatenate/1 -> Xb/1
  [alpha] -> "Tension from UAV, X and r directions"/1(alpha)
  [XZb] -> Delay3/1
  [XZu_dot] -> Delay4/1
  [XZb_dot] -> Delay5/1
  [XZu_ddot] -> Delay6/1
  [XZb_ddot] -> Delay8/1
  [alpha_ddot] -> Gain2/1
  Delay4/1 -> azimuthal dynamics/4("Xu_dot ")
  [X123_ddot] -> Delay9/1
  Delay5/1 -> azimuthal dynamics/5(Xb_dot)
  Delay6/1 -> azimuthal dynamics/6(Xu_ddot)
  Delay8/1 -> azimuthal dynamics/7("Xb_ddot   ")
  Delay9/1 -> azimuthal dynamics/8("X123_ddot  ")
  [coupled] -> Delay1/1
  Delay1/1 -> V_im 1/1, azimuthal dynamics/1(coupled)
  Delay11/1 -> Quadrotor Dynamics Outer-Loop/1(X123)
  Delay12/1 -> Quadrotor Dynamics Outer-Loop/3(Xddot123)
  Delay7/1 -> Quadrotor Dynamics Outer-Loop/2(Xdot123)
  Delay13/1 -> Quadrotor Dynamics Outer-Loop/4(coupled)
  azimuthal dynamics/6(r dot) -> "  rdot"/1, [rr_dot]
  azimuthal dynamics/7(r ddot) -> "  rddot"/1, [rr_ddot]
  "Tension from UAV, X and r directions"/2("T, from uav z") -> Coupling state/1(pos_T), Cable Tension/1, Vector Concatenate10/2
  [re_couple] -> Coupling state/2(re_couple)
  Coupling state/1(is coupled) -> "is coupled "/1, coupled/1, [coupled]
  Quadrotor Dynamics Outer-Loop/3(ddot(Xu)) -> Xu_ddot/1, theta u1/1, [XZu_ddot]
  Quadrotor Dynamics Outer-Loop/4(acc_b_u) -> Terminator/1
  "Tension from UAV, X and r directions"/1("T, from r") -> Vector Concatenate10/1
  D_u (vector for simplification)/1(Du) -> Product1/1
  [XZu_dot] -> Sum6/2
  Sum6/1 -> D_u (vector for simplification)/1(Vr), Product1/2
  Delay2/1 -> Quadrotor Dynamics Outer-Loop/7(Du)
  V_wind/1 -> Delay10/1
  Delay10/1 -> Sum6/1

== system Marine_LocoMotive_UAV_est_git/Save to file/mean absolute error ==
  In1 : Inport
  Abs : Abs
  Add : Sum
  Constant : Constant  Value=T
  Delay : Delay  DelayLength=1
  IC : InitialCondition
  Product1 : Product  Inputs=*/
  Product2 : Product  Inputs=*/
  Out1 : Outport
  wires:
  Product2/1 -> IC/1
  Add/1 -> Product1/1, Delay/1
  Delay/1 -> Add/1
  [time] -> Product2/1
  In1/1 -> Abs/1
  Product1/1 -> Out1/1
  Constant/1 -> Product2/2
  IC/1 -> Product1/2
  Abs/1 -> Add/2

== system Marine_LocoMotive_UAV_est_git/Scope/Subsystem ==
  In1 : Inport
  In2 : Inport  Port=2
  Product : Product
  Sqrt : Sqrt  SaturateOnIntegerOverflow=on
  Subtract : Sum  Inputs=+-
  Sum of Elements : Sum  Inputs=+
  Out1 : Outport
  wires:
  In1/1 -> Subtract/2
  Product/1 -> Sum of Elements/1
  Subtract/1 -> Product/2, Product/1
  In2/1 -> Subtract/1
  Sqrt/1 -> Out1/1, [r]
  Sum of Elements/1 -> Sqrt/1

== system Marine_LocoMotive_UAV_est_git/Scope/absolute mean ==
  u : Inport
  Abs : Abs
  Bias : Bias  Bias=1/1000
  Clock : Clock
  Current velocity : Scope
  Current velocity1 : Scope
  Current velocity2 : Scope
  Discrete-Time Integrator : DiscreteIntegrator  gainval=1  SampleTime=T  ICPrevOutput=DiscIntNeverNeededParam  ICPrevScaledInput=DiscIntNeverNeededParam
  Divide1 : Product  Inputs=*/
  mean : Outport
  wires:
  Discrete-Time Integrator/1 -> Current velocity1/1, Divide1/1
  Abs/1 -> Discrete-Time Integrator/1
  u/1 -> Current velocity/1, Abs/1
  Divide1/1 -> mean/1
  Clock/1 -> Bias/1
  Bias/1 -> Current velocity2/1, Divide1/2

== system Marine_LocoMotive_UAV_est_git/Scope/absolute mean1 ==
  u : Inport
  Abs : Abs
  Bias : Bias  Bias=1/1000
  Clock : Clock
  Current velocity : Scope
  Current velocity1 : Scope
  Current velocity2 : Scope
  Discrete-Time Integrator : DiscreteIntegrator  gainval=1  SampleTime=T  ICPrevOutput=DiscIntNeverNeededParam  ICPrevScaledInput=DiscIntNeverNeededParam
  Divide1 : Product  Inputs=*/
  mean : Outport
  wires:
  Clock/1 -> Bias/1
  Divide1/1 -> mean/1
  u/1 -> Abs/1, Current velocity/1
  Abs/1 -> Discrete-Time Integrator/1
  Discrete-Time Integrator/1 -> Divide1/1, Current velocity1/1
  Bias/1 -> Divide1/2, Current velocity2/1

== system Marine_LocoMotive_UAV_est_git/Sea2/Single Wave ==
  note: Aw.Sin
  time : Inport
  x(t) : Inport  Port=2
  Constant : Constant  Value=epsilon
  Gain : Gain  Gain=omega
  Gain1 : Gain  Gain=k
  Gain2 : Gain  Gain=A
  Gain3 : Gain  Gain=omega*A
  Gain4 : Gain  Gain=omega*A
  Gain5 : Gain  Gain=A*k
  Sum : Sum  Inputs=++-
  Trigonometric Function : Trigonometry  Operator=sincos
  Trigonometric Function1 : Trigonometry  Operator=atan
  direction : Gain  Gain=w_dir
  direction1 : Gain  Gain=w_dir
  direction2 : Gain  Gain=w_dir
  zeta(x,t) : Outport
  theta_w(x,t) : Outport  Port=2
  u(z0,x,t) : Outport  Port=3
  w(z0,x,t) : Outport  Port=4
  wires:
  Gain/1 -> Sum/2
  Gain1/1 -> Sum/3
  x(t)/1 -> Gain1/1
  Trigonometric Function/1 -> Gain3/1, Gain2/1
  Constant/1 -> Sum/1
  time/1 -> direction/1
  direction/1 -> Gain/1
  Gain2/1 -> zeta(x,t)/1  "zeta(x,t)"
  Trigonometric Function/2 -> Gain5/1, Gain4/1
  Sum/1 -> Trigonometric Function/1
  Trigonometric Function1/1 -> theta_w(x,t)/1
  Gain5/1 -> Trigonometric Function1/1
  Gain3/1 -> direction1/1
  Gain4/1 -> direction2/1
  direction1/1 -> u(z0,x,t)/1
  direction2/1 -> w(z0,x,t)/1

== system Marine_LocoMotive_UAV_est_git/Sea2/Single Wave1 ==
  note: Aw.Sin
  time : Inport
  x(t) : Inport  Port=2
  Constant : Constant  Value=epsilon
  Gain : Gain  Gain=omega
  Gain1 : Gain  Gain=k
  Gain2 : Gain  Gain=A
  Gain3 : Gain  Gain=omega*A
  Gain4 : Gain  Gain=omega*A
  Gain5 : Gain  Gain=A*k
  Sum : Sum  Inputs=++-
  Trigonometric Function : Trigonometry  Operator=sincos
  Trigonometric Function1 : Trigonometry  Operator=atan
  direction : Gain  Gain=w_dir
  direction1 : Gain  Gain=w_dir
  direction2 : Gain  Gain=w_dir
  zeta(x,t) : Outport
  theta_w(x,t) : Outport  Port=2
  u(z0,x,t) : Outport  Port=3
  w(z0,x,t) : Outport  Port=4
  wires:
  direction2/1 -> w(z0,x,t)/1
  direction1/1 -> u(z0,x,t)/1
  Gain4/1 -> direction2/1
  Gain3/1 -> direction1/1
  Gain5/1 -> Trigonometric Function1/1
  Trigonometric Function1/1 -> theta_w(x,t)/1
  Sum/1 -> Trigonometric Function/1
  Trigonometric Function/2 -> Gain4/1, Gain5/1
  Gain2/1 -> zeta(x,t)/1  "zeta(x,t)"
  direction/1 -> Gain/1
  time/1 -> direction/1
  Constant/1 -> Sum/1
  Trigonometric Function/1 -> Gain2/1, Gain3/1
  x(t)/1 -> Gain1/1
  Gain1/1 -> Sum/3
  Gain/1 -> Sum/2

== system Marine_LocoMotive_UAV_est_git/Sea2/Theta_water surface (two waves) ==
  w1 : Inport
  w2 : Inport  Port=2
  Gain2 : Gain  Gain=1/(omega_w)
  Gain3 : Gain  Gain=k_w
  Gain4 : Gain  Gain=1/(omega_w2)
  Gain5 : Gain  Gain=k_w2
  Sum2 : Sum  Inputs=++|
  direction1 : Gain  Gain=1/w_dir
  direction2 : Gain  Gain=1/w_dir2
  Out1 : Outport
  wires:
  Gain4/1 -> direction2/1
  direction2/1 -> Gain5/1
  Sum2/1 -> Out1/1
  w1/1 -> Gain2/1
  Gain3/1 -> Sum2/1
  Gain5/1 -> Sum2/2
  w2/1 -> Gain4/1
  direction1/1 -> Gain3/1
  Gain2/1 -> direction1/1

== system Marine_LocoMotive_UAV_est_git/Sensors and Filters/Coupling detection by r ==
  In1 : Inport
  In2 : Inport  Port=2
  Constant1 : Constant  Value=0
  Coupling state : Subsystem
  Data Type Conversion : DataTypeConversion  OutDataTypeStr=double
  IC2 : InitialCondition  Value=0
  Switch14 : Switch  Criteria=u2 > Threshold  Threshold=0.5
  cable length with safety margine : simulink/Logic and Bit Operations/Compare To Constant  relop=>=  const=Lc_0+0.005  OutDataTypeStr=boolean
  is coupled {,2..4} (4 alike) : Scope
  is coupled : Outport
  wires:
  IC2/1 -> Switch14/3
  In1/1 -> is coupled 3/1, Coupling state/1(r_est), is coupled 2/1, cable length with safety margine/1
  Switch14/1 -> [re_couple]
  cable length with safety margine/1 -> is coupled 4/1, Data Type Conversion/1
  [re_couple] -> Coupling state/2(re_couple)
  Data Type Conversion/1 -> IC2/1
  Coupling state/1(is coupled) -> is coupled/1, "is coupled "/1
  Constant1/1 -> Switch14/1
  In2/1 -> Switch14/2

== system Marine_LocoMotive_UAV_est_git/Sensors and Filters/Data processing ==
  Acc : Inport
  "GPS " : Inport  Port=2
  p,q,r : Inport  Port=3
  Sonar : Inport  Port=4
  Estimate Attitude : Subsystem  TreatAsAtomicUnit=on  SystemSampleTime=Tc
  Estimate Position : Subsystem  TreatAsAtomicUnit=on  SystemSampleTime=Tc
  "Euler " : Selector  InputPortWidth=5  IndexOptions=Index vector (dialog)  Indices=[3]  OutputSizes=1
  GPS : InportShadow  Port=2
  Xe_est : Outport
  Ve_est : Outport  Port=2
  q_gyro : Outport  Port=3
  "q_est " : Outport  Port=4
  pitch_est : Outport  Port=5
  wires:
  GPS/1 -> "Euler "/1
  Acc/1 -> Estimate Attitude/1(Acc)
  p,q,r/1 -> Estimate Attitude/2(q)
  "Euler "/1 -> Estimate Attitude/3(Euler)
  Estimate Attitude/2(q_f) -> "q_est "/1
  "GPS "/1 -> Estimate Position/1(OptiTrack)
  Estimate Position/1(Xe) -> Xe_est/1
  Estimate Position/2(Ve) -> Ve_est/1
  Estimate Attitude/1(q_g) -> q_gyro/1
  Sonar/1 -> Estimate Position/3(Sonar)
  Estimate Attitude/3(" pitch") -> Estimate Position/2("pitch, Kalman"), pitch_est/1

== system Marine_LocoMotive_UAV_est_git/Sensors and Filters/GPS//INS ==
  X : Inport
  X_dot : Inport  Port=2
  X_ddot : Inport  Port=3
  q : Inport  Port=4
  theta : Inport  Port=5
  Discrete Derivative1 : simulink/Discrete/Discrete Derivative  gainval=1.0  ICPrevScaledInput=0.0  OutMin=[]  OutMax=[]  OutDataType=fixdt(1, 16)  OutScaling=2^-10  DoSatur=off
  Discrete Derivative2 : simulink/Discrete/Discrete Derivative  gainval=1.0  ICPrevScaledInput=0.0  OutMin=[]  OutMax=[]  OutDataType=fixdt(1, 16)  OutScaling=2^-10  DoSatur=off
  GPS noise : RandomNumber  Variance=5/10000  Seed=123  SampleTime=Tg
  Gain : Gain  Gain=0.25
  Gain1 : Gain  Gain=0.5
  Gain2 : Gain
  Gain3 : Gain
  Gain4 : Gain
  IMU noise : RandomNumber  Variance=1/10000  Seed=2235  SampleTime=Ts
  Low Pass Filter{1,3..5} (4 alike) : DiscreteTransferFcn  Numerator=Bm_LPF2  Denominator=Am_LPF2
  Low Pass Filter2 : DiscreteTransferFcn  Numerator=Bm_LPF  Denominator=Am_LPF
  Mux4 : Mux  Inputs=2
  Rate Transition : RateTransition
  Rate Transition1 : RateTransition
  Sum{1,3..6} (5 alike) : Sum  Inputs=++|
  q1 : Scope
  q2 : Scope
  q3 : Scope
  X_est : Outport
  X_dot_est : Outport  Port=2
  q_est : Outport  Port=3
  theta_est : Outport  Port=4
  X_ddot_est : Outport  Port=5
  wires:
  Sum4/1 -> X_dot_est/1
  Low Pass Filter1/1 -> Low Pass Filter3/1
  Gain3/1 -> Sum6/1
  q/1 -> Sum6/2
  theta/1 -> Sum5/2
  Gain2/1 -> Sum5/1
  Rate Transition1/1 -> Low Pass Filter2/1
  IMU noise/1 -> Rate Transition1/1
  Mux4/1 -> Gain1/1
  X/1 -> Sum3/2
  GPS noise/1 -> Rate Transition/1
  Rate Transition/1 -> Low Pass Filter1/1
  Sum5/1 -> theta_est/1
  X_dot/1 -> Sum4/2
  Sum3/1 -> X_est/1
  Sum6/1 -> q_est/1
  Low Pass Filter2/1 -> Gain3/1, Gain2/1, q2/1
  Low Pass Filter3/1 -> Mux4/2, Mux4/1
  Discrete Derivative1/1 -> Low Pass Filter4/1
  Gain1/1 -> Discrete Derivative1/1, Sum3/1, q1/1
  Gain/1 -> Discrete Derivative2/1, Sum4/1, q3/1
  Discrete Derivative2/1 -> Low Pass Filter5/1
  X_ddot/1 -> Sum1/2
  Gain4/1 -> Sum1/1
  Sum1/1 -> X_ddot_est/1
  Low Pass Filter4/1 -> Gain/1
  Low Pass Filter5/1 -> Gain4/1

== system Marine_LocoMotive_UAV_est_git/Sensors and Filters/Sensors ==
  note: Gyro noise destroys the estimation
  note: Acc noise does not affect estimation
  "q " : Inport
  Ab : Inport  Port=2
  Xe : Inport  Port=3
  Euler : Inport  Port=4
  " Sonar (10Hz) (true elevation instead real sonar signal)" : Subsystem
  Accelerometer (500Hz) : Subsystem  TreatAsAtomicUnit=on  SystemSampleTime=Ts
  "GPS (10Hz) " : Subsystem  TreatAsAtomicUnit=on  SystemSampleTime=Tg
  Gyro (500Hz) : Subsystem  TreatAsAtomicUnit=on  SystemSampleTime=Ts
  RT : RateTransition  OutPortSampleTime=Ts
  Rate Transition : RateTransition
  Rate Transition1 : RateTransition
  Rate Transition2 : RateTransition  Deterministic=off  InitialCondition=[X0_u Theta0 1 1]
  Z : Selector  InputPortWidth=5  IndexOptions=Index vector (dialog)  Indices=2  OutputSizes=1
  acc : Scope  Commented=on
  pqr : Scope  Commented=on
  rotation matrix R : Subsystem
  Acc : Outport
  GPS : Outport  Port=2
  " q" : Outport  Port=3
  Sonar : Outport  Port=4
  wires:
  Xe/1 -> "GPS (10Hz) "/1(Xe)
  Ab/1 -> RT/1
  "q "/1 -> Gyro (500Hz)/1(q)
  Euler/1 -> rotation matrix R/1(angle (rad)), "GPS (10Hz) "/2(Euler)
  Accelerometer (500Hz)/1(Acc) -> Rate Transition1/1
  Gyro (500Hz)/1(" q") -> Rate Transition/1
  Z/1 -> " Sonar (10Hz) (true elevation instead real sonar signal)"/1(sonar (m))
  " Sonar (10Hz) (true elevation instead real sonar signal)"/1(calib sonar (m)) -> Sonar/1
  Rate Transition/1 -> pqr/1, " q"/1
  Rate Transition1/1 -> acc/1, Acc/1
  RT/1 -> Accelerometer (500Hz)/1(Ab)
  rotation matrix R/1(R) -> "GPS (10Hz) "/3(DCM_b2e)
  Rate Transition2/1 -> Z/1, GPS/1
  "GPS (10Hz) "/1(GPS) -> Rate Transition2/1

== system Marine_LocoMotive_UAV_est_git/Sensors and Filters/Sterio camera + encoder ==
  note: the error in alpha should relate to the stereo camera accuracy and the radial distance:
      | alpha = atan( 2cm / 7 m) = 0.0029 rad.
  alpha : Inport
  alpha_dot : Inport  Port=2
  alpha_ddot : Inport  Port=3
  r : Inport  Port=4
  r_dot : Inport  Port=5
  r_ddot : Inport  Port=6
  Discrete Derivative{,1..3} (4 alike) : simulink/Discrete/Discrete Derivative  gainval=1.0  ICPrevScaledInput=0.0  OutMin=[]  OutMax=[]  OutDataType=fixdt(1, 16)  OutScaling=2^-10  DoSatur=off
  Gain1 : Gain  Gain=0.5
  Gain2 : Gain  Gain=0.3
  Gain4 : Gain
  Gain5 : Gain
  Gain6 : Gain  Gain=0.25
  Gain7 : Gain  Gain=0.5
  Low Pass Filter{1..9} (9 alike) : DiscreteTransferFcn  Numerator=Bm_LPF2  Denominator=Am_LPF2
  Low Pass Filter10 : DiscreteTransferFcn  Commented=on  Numerator=Bm_LPF2  Denominator=Am_LPF2
  Low Pass Filter11 : DiscreteTransferFcn  Commented=on  Numerator=Bm_LPF2  Denominator=Am_LPF2
  Rate Transition1 : RateTransition
  Rate Transition2 : RateTransition
  Sum{1..2,7..10} (6 alike) : Sum  Inputs=++|
  stereo cam noise (location in frame) : RandomNumber  Variance=1/100000  Seed=5684  SampleTime=Tsc
  sterio cam noise (range) : RandomNumber  Variance=1/1000  Seed=1142  SampleTime=Tsc
  alpha_est : Outport
  alpha_dot_est : Outport  Port=2
  r_est : Outport  Port=3
  r_dot_est : Outport  Port=4
  alpha_ddot_est : Outport  Port=5
  r_ddot_est : Outport  Port=6
  wires:
  Rate Transition2/1 -> Low Pass Filter3/1
  stereo cam noise (location in frame)/1 -> Rate Transition2/1
  Gain5/1 -> Sum8/1
  Sum10/1 -> r_dot_est/1
  Discrete Derivative/1 -> Low Pass Filter8/1
  alpha_dot/1 -> Sum9/2
  Gain4/1 -> Sum7/1
  Discrete Derivative1/1 -> Low Pass Filter7/1
  Sum7/1 -> alpha_est/1
  Sum8/1 -> r_est/1
  r/1 -> Sum8/2
  alpha/1 -> Sum7/2
  r_dot/1 -> Sum10/2
  Sum9/1 -> alpha_dot_est/1
  sterio cam noise (range)/1 -> Rate Transition1/1
  Rate Transition1/1 -> Low Pass Filter1/1
  Sum1/1 -> alpha_ddot_est/1
  Discrete Derivative2/1 -> Low Pass Filter6/1
  Gain6/1 -> Discrete Derivative2/1, Sum9/1
  Gain1/1 -> Sum1/1
  alpha_ddot/1 -> Sum1/2
  r_ddot/1 -> Sum2/2
  Discrete Derivative3/1 -> Low Pass Filter9/1
  Gain2/1 -> Sum2/1
  Sum2/1 -> r_ddot_est/1
  Gain7/1 -> Discrete Derivative3/1, Sum10/1
  Low Pass Filter2/1 -> Gain7/1
  Low Pass Filter4/1 -> Gain2/1
  Low Pass Filter5/1 -> Gain6/1
  Low Pass Filter6/1 -> Gain1/1
  Low Pass Filter7/1 -> Low Pass Filter5/1
  Low Pass Filter8/1 -> Low Pass Filter2/1
  Low Pass Filter9/1 -> Low Pass Filter4/1
  Low Pass Filter3/1 -> Gain4/1, Discrete Derivative1/1
  Low Pass Filter1/1 -> Gain5/1, Discrete Derivative/1

== system Marine_LocoMotive_UAV_est_git/Sensors and Filters/quadrotor position from relative buoy-UAV position ==
  X_u : Inport
  Xdot_u : Inport  Port=2
  Xddot_u : Inport  Port=3
  r : Inport  Port=4
  r_dot : Inport  Port=5
  r_ddot : Inport  Port=6
  alpha : Inport  Port=7
  alpha_dot : Inport  Port=8
  alpha_ddot : Inport  Port=9
  Demux : Demux  Outputs=2
  Gain1 : Gain  Gain=-1
  Gain2 : Gain  Gain=2
  Product1 : Product  Inputs=3
  Product{2,4..5,7..8} (5 alike) : Product
  Product3 : Product  Multiplication=Matrix(*)
  Product6 : Product  Multiplication=Matrix(*)
  Sum : Sum  Inputs=|+-
  Sum1 : Sum  Inputs=|+-
  Sum2 : Sum  Inputs=+-|
  Sum3 : Sum  Inputs=++|
  Sum4 : Sum  Inputs=+-|
  Trigonometric Function : Trigonometry  Operator=sincos
  Vector Concatenate{1..4} (4 alike) : Concatenate
  r1 : InportShadow  Port=4
  r_dot1 : InportShadow  Port=5
  "rotation matrix R " : Subsystem
  theta u{1..2,4,6} (4 alike) : Scope
  Xb : Outport
  Xdot_b : Outport  Port=2
  Xddot_b : Outport  Port=3
  wires:
  Trigonometric Function/2 -> Product5/1
  Trigonometric Function/1 -> Product4/1
  alpha/1 -> "rotation matrix R "/1(angle (rad)), Trigonometric Function/1  "alpha"
  Sum1/1 -> Vector Concatenate3/2
  Vector Concatenate3/1 -> theta u4/1, Xb/1
  Product5/1 -> Sum/2
  Demux/2 -> Sum1/1  "z_u"
  Product4/1 -> Sum1/2
  Sum/1 -> Vector Concatenate3/1
  X_u/1 -> Demux/1
  Demux/1 -> Sum/1  "x_u"
  Vector Concatenate2/1 -> Product3/2
  Sum4/1 -> Xdot_b/1, theta u6/1
  Product3/1 -> Sum4/2
  r/1 -> Product2/1, Product5/2, Product4/2
  r_dot/1 -> theta u1/1, Vector Concatenate2/1
  Product2/1 -> theta u2/1, Vector Concatenate2/2
  alpha_dot/1 -> Product2/2, Product7/1, Product1/2, Product1/1
  Xdot_u/1 -> Sum4/1
  Product6/1 -> Sum2/2
  Gain2/1 -> Vector Concatenate1/2
  "rotation matrix R "/1(R) -> Product6/1, Product3/1
  Product1/1 -> Gain1/1
  Sum3/1 -> Product6/2
  r1/1 -> Product8/1, Product1/3
  Product7/1 -> Gain2/1
  r_dot1/1 -> Product7/2
  Xddot_u/1 -> Sum2/1
  Vector Concatenate1/1 -> Sum3/2
  r_ddot/1 -> Vector Concatenate4/1
  Product8/1 -> Vector Concatenate4/2
  alpha_ddot/1 -> Product8/2
  Vector Concatenate4/1 -> Sum3/1
  Gain1/1 -> Vector Concatenate1/1
  Sum2/1 -> Xddot_b/1

== system Marine_LocoMotive_UAV_est_git/UAV controller/Coupling ==
  U1 : Inport
  U3 : Inport  Port=2
  Coupling : Subsystem
  sat : Subsystem
  u_1 : Outport
  theta_d : Outport  Port=2
  wires:
  Coupling/1(u1 (N)) -> u_1/1
  Coupling/2(phi_d (rad)) -> sat/1(u)
  U3/1 -> Coupling/2(U3)
  U1/1 -> Coupling/1(U1)
  sat/1(sat(u)) -> theta_d/1

== system Marine_LocoMotive_UAV_est_git/UAV controller/Coupling  ==
  u_T : Inport
  u_a : Inport  Port=2
  alpha : Inport  Port=3
  theta_q : Inport  Port=4
  Add5 : Sum  Inputs=2
  Bias : Bias  Bias=-pi/2
  Product1 : Product
  Product3 : Product
  Saturation : Saturate  UpperLimit=LIMIT_uCMD_HEIGHT  LowerLimit=m_u*g*0.5
  Scope{,1..6} (7 alike) : Scope
  Sqrt : Sqrt  SaturateOnIntegerOverflow=on
  Subsystem2 : Subsystem  Commented=on
  Subsystem3 : Subsystem  Commented=on
  Subtract : Sum  Inputs=--
  Trigonometric Function1 : Trigonometry  Operator=atan2
  Vector Concatenate : Concatenate
  alpha1 : InportShadow  Port=3
  "sat " : Subsystem
  u_T switch : Subsystem
  u_a switch : Subsystem
  u1 : Outport
  theta_c : Outport  Port=2
  wires:
  Bias/1 -> Scope2/1, Subtract/1
  Product1/1 -> Add5/1, Scope/1
  Sqrt/1 -> Saturation/1
  Subtract/1 -> "sat "/1(u)
  Trigonometric Function1/1 -> Scope4/1, Subtract/2
  Product3/1 -> Scope1/1, Add5/2
  Add5/1 -> Sqrt/1
  alpha/1 -> Bias/1
  Saturation/1 -> Scope6/1, u1/1
  "sat "/1(sat(u)) -> Scope3/1, [theta_c], theta_c/1
  u_a/1 -> Vector Concatenate/1, Trigonometric Function1/1, u_a switch/1(u_a)
  u_T switch/1(u_T_out) -> Product1/2, Product1/1
  Vector Concatenate/1 -> Scope5/1
  alpha1/1 -> u_a switch/2(alpha), u_T switch/1(alpha)
  theta_q/1 -> u_a switch/3(theta_q), u_T switch/2(theta_q)
  u_T/1 -> Vector Concatenate/2, Trigonometric Function1/2, u_T switch/3(u_T)
  u_a switch/1(u_a_out) -> Product3/1, Product3/2

== system Marine_LocoMotive_UAV_est_git/UAV controller/Enabled Subsystem1 ==
  u : Inport
  reset : Inport  Port=2
  u0 : Inport  Port=3
  Enable : EnablePort
  Logical Operator : Logic  Operator=NOT  AllPortsSameDT=off  OutDataTypeStr=boolean
  Low Pass Filter5 : DiscreteTransferFcn  Numerator=Bm_rdeL_LPF  Denominator=Am_rdeL_LPF  InitialStatesSource=Input port  ExternalReset=Level
      settings: InputPortMap=u0,r7,p5
  Mux2 : Mux  Inputs=2
  adjustment for this specific transfer function : Gain  Gain=84.6505602
  r_dot filt : Scope
  r_dot filt1 : Scope
  y : Outport
  wires:
  u/1 -> Mux2/2, Low Pass Filter5/1
  Low Pass Filter5/1 -> Mux2/1, y/1
  Logical Operator/1 -> r_dot filt1/1, Low Pass Filter5/2
  u0/1 -> adjustment for this specific transfer function/1
  Mux2/1 -> r_dot filt/1
  adjustment for this specific transfer function/1 -> Low Pass Filter5/3
  reset/1 -> Logical Operator/1

== system Marine_LocoMotive_UAV_est_git/UAV controller/V controller ==
  V_bar : Inport
  V : Inport  Port=2
  Discrete Derivative1 : simulink/Discrete/Discrete Derivative  gainval=1.0  ICPrevScaledInput=0.0  OutMin=[]  OutMax=[]  OutDataType=fixdt(1, 16)  OutScaling=2^-10  DoSatur=off
  Discrete Derivative6 : simulink/Discrete/Discrete Derivative  gainval=1.0  ICPrevScaledInput=0.0  OutMin=[]  OutMax=[]  OutDataType=fixdt(1, 16)  OutScaling=2^-10  DoSatur=off
  Discrete-Time Integrator : DiscreteIntegrator  SampleTime=-1  LimitOutput=on  UpperSaturationLimit=300  LowerSaturationLimit=-200  ICPrevOutput=DiscIntNeverNeededParam  ICPrevScaledInput=DiscIntNeverNeededParam
  Gain : Gain  Gain=ki_x
  IC : InitialCondition  Value=0
  IC1 : InitialCondition  Value=0
  IC2 : InitialCondition  Value=0
  K1 : Gain  Gain=kp_x
  K2 : Gain  Gain=kd_x
  K3 : Gain
  K4 : Gain
  Mux : Mux  Inputs=2
  Mux1 : Mux  Inputs=2
  Product : Product
  Saturation1 : Saturate  UpperLimit=50  LowerLimit=-20
  Scope{1..6} (6 alike) : Scope
  Step : Step  Time=3*T  SampleTime=0
  Sum : Sum  Inputs=|+-
  Sum1 : Sum  Inputs=|+-
  Sum4 : Sum  Inputs=---
  U1 (m/s^2) : Outport
  wires:
  Sum1/1 -> Product/1  "ev"
  Sum/1 -> Discrete-Time Integrator/1, K1/1  "ex"
  V_bar/1 -> Mux/2, Sum/2, Discrete Derivative6/1
  Sum4/1 -> Saturation1/1
  K1/1 -> K4/1
  K2/1 -> K3/1
  Discrete-Time Integrator/1 -> Gain/1
  Gain/1 -> Scope3/1, Sum4/3
  Saturation1/1 -> Scope4/1, U1 (m/s^2)/1
  Mux/1 -> Scope1/1
  Discrete Derivative1/1 -> IC1/1
  Mux1/1 -> Scope2/1
  Discrete Derivative6/1 -> IC2/1
  IC/1 -> Discrete Derivative1/1, Mux/1, Sum/1
  V/1 -> IC/1
  IC1/1 -> Sum1/1, Mux1/1
  IC2/1 -> Mux1/2, Sum1/2
  K3/1 -> Scope5/1, Sum4/2
  K4/1 -> Scope6/1, Sum4/1
  Product/1 -> K2/1
  Step/1 -> Product/2
